simulink model "power_wind"  (R2014b)
settings: Solver=ode23tb  StartTime=0.0  StopTime=20  MaxStep=1/60  RelTol=1e-4  AbsTol=1e-3
InitFcn:
  | xInitial = init_power_wind_ig;
undefined symbols (not defined in the file): D1, D11, Delta
libraries: powerlib_meascontrol x45, powerlib x29, DRlib x3, factslib x1
(part 3 of 4)

== system power_wind/Wind Farm/Wind Turbine Protections/Protection System3/AC Voltage Protection/Voltage Measurement/magnitude1 ==
  In1 : Inport
  Complex to Real-Imag : ComplexToRealImag
  Fourier1 : Subsystem  mask(Fourier analyser){f1=Freq, n=0}
      mask prompts: f1 "Fundamental frequency f1 (Hz):"; n "Harmonic n (0=DC; 1=fundamental; 2=2nd harm;  ...) :"
      mask help: The Fourier block performs a Fourier analysis of the input signal over a running window of one cycle of the fundamental frequency. First and second outputs return respectively the magnitude and phase (degrees) of the harmonic component specified.
      mask init:
      | k=2-(n==0);
      mask Help: helpview(psbhelp)
  Fourier2 : Subsystem  mask(Fourier analyser){f1=Freq, n=0}
      mask prompts: f1 "Fundamental frequency f1 (Hz):"; n "Harmonic n (0=DC; 1=fundamental; 2=2nd harm;  ...) :"
      mask help: The Fourier block performs a Fourier analysis of the input signal over a running window of one cycle of the fundamental frequency. First and second outputs return respectively the magnitude and phase (degrees) of the harmonic component specified.
      mask init:
      | k=2-(n==0);
      mask Help: helpview(psbhelp)
  Math Function : Math  Operator=hypot  SaturateOnIntegerOverflow=on
  Terminator : Terminator
  Terminator1 : Terminator
  Out1 : Outport
  wires:
  Complex to Real-Imag/1 -> Fourier1/1(signal)
  Complex to Real-Imag/2 -> Fourier2/1(signal)
  Fourier1/2(angle) -> Terminator/1
  Fourier2/2(angle) -> Terminator1/1
  Fourier1/1(magnitude) -> Math Function/1
  Fourier2/1(magnitude) -> Math Function/2
  Math Function/1 -> Out1/1
  In1/1 -> Complex to Real-Imag/1

== system power_wind/Wind Farm/Wind Turbine Protections/Protection System3/AC Voltage Protection/Voltage Measurement/magnitude2 ==
  In1 : Inport
  Complex to Real-Imag : ComplexToRealImag
  Fourier1 : Subsystem  mask(Fourier analyser){f1=Freq, n=0}
      mask prompts: f1 "Fundamental frequency f1 (Hz):"; n "Harmonic n (0=DC; 1=fundamental; 2=2nd harm;  ...) :"
      mask help: The Fourier block performs a Fourier analysis of the input signal over a running window of one cycle of the fundamental frequency. First and second outputs return respectively the magnitude and phase (degrees) of the harmonic component specified.
      mask init:
      | k=2-(n==0);
      mask Help: helpview(psbhelp)
  Fourier2 : Subsystem  mask(Fourier analyser){f1=Freq, n=0}
      mask prompts: f1 "Fundamental frequency f1 (Hz):"; n "Harmonic n (0=DC; 1=fundamental; 2=2nd harm;  ...) :"
      mask help: The Fourier block performs a Fourier analysis of the input signal over a running window of one cycle of the fundamental frequency. First and second outputs return respectively the magnitude and phase (degrees) of the harmonic component specified.
      mask init:
      | k=2-(n==0);
      mask Help: helpview(psbhelp)
  Math Function : Math  Operator=hypot  SaturateOnIntegerOverflow=on
  Terminator : Terminator
  Terminator1 : Terminator
  Out1 : Outport
  wires:
  In1/1 -> Complex to Real-Imag/1
  Math Function/1 -> Out1/1
  Fourier2/1(magnitude) -> Math Function/2
  Fourier1/1(magnitude) -> Math Function/1
  Fourier2/2(angle) -> Terminator1/1
  Fourier1/2(angle) -> Terminator/1
  Complex to Real-Imag/2 -> Fourier2/1(signal)
  Complex to Real-Imag/1 -> Fourier1/1(signal)

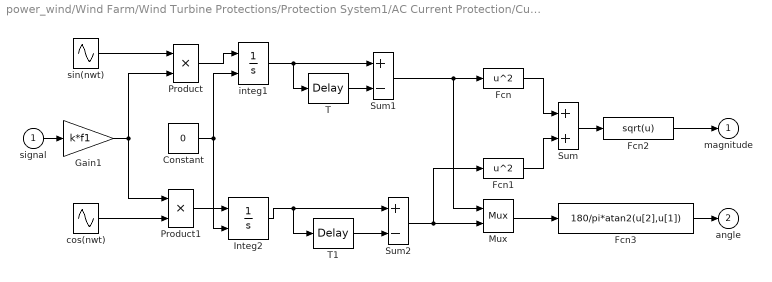
== system power_wind/Wind Farm/Wind Turbine Protections/Protection System1/AC Current Protection/Current Measurement/magnitude/Fourier1 ==
  signal : Inport
  Constant : Constant  Value=0
  Fcn : Fcn  Expr=u^2
  Fcn1 : Fcn  Expr=u^2
  Fcn2 : Fcn  Expr=sqrt(u)
  Fcn3 : Fcn  Expr=180/pi*atan2(u[2],u[1])
  Gain1 : Gain  Gain=k*f1  SaturateOnIntegerOverflow=on  OutDataTypeStr=Inherit: Same as input  ParamDataTypeStr=Inherit: Same as input
  Integ2 : Integrator  InitialConditionSource=external
  Mux : Mux  Inputs=2
  Product : Product  SaturateOnIntegerOverflow=on  InputSameDT=on  OutDataTypeStr=Inherit: Same as first input
  Product1 : Product  SaturateOnIntegerOverflow=on  InputSameDT=on  OutDataTypeStr=Inherit: Same as first input
  Sum : Sum  SaturateOnIntegerOverflow=on  InputSameDT=on  OutDataTypeStr=Inherit: Same as first input
  Sum1 : Sum  Inputs=+-  SaturateOnIntegerOverflow=on  InputSameDT=on  OutDataTypeStr=Inherit: Same as first input
  Sum2 : Sum  Inputs=+-  SaturateOnIntegerOverflow=on  InputSameDT=on  OutDataTypeStr=Inherit: Same as first input
  T : TransportDelay  DelayTime=1/f1  BufferSize=2048
  T1 : TransportDelay  DelayTime=1/f1  BufferSize=2048
  cos(nwt) : Sin  Frequency=2*pi*n*f1  Phase=pi/2  SampleTime=0
  integ1 : Integrator  InitialConditionSource=external
  sin(nwt) : Sin  Frequency=2*pi*n*f1  SampleTime=0
  magnitude : Outport  InitialOutput=0
  angle : Outport  Port=2  InitialOutput=0
  wires:
  Constant/1 -> integ1/2, Integ2/2
  Sum/1 -> Fcn2/1
  Fcn/1 -> Sum/1
  Fcn1/1 -> Sum/2
  Mux/1 -> Fcn3/1
  Fcn3/1 -> angle/1
  sin(nwt)/1 -> Product/1
  cos(nwt)/1 -> Product1/2
  Product/1 -> integ1/1
  Product1/1 -> Integ2/1
  T/1 -> Sum1/2
  T1/1 -> Sum2/2
  integ1/1 -> Sum1/1, T/1
  Integ2/1 -> T1/1, Sum2/1
  Sum2/1 -> Fcn1/1, Mux/2
  Sum1/1 -> Fcn/1, Mux/1
  signal/1 -> Gain1/1
  Gain1/1 -> Product/2, Product1/1
  Fcn2/1 -> magnitude/1

== system power_wind/Wind Farm/Wind Turbine Protections/Protection System1/AC Current Protection/Current Measurement/magnitude/Fourier2 ==
  signal : Inport
  Constant : Constant  Value=0
  Fcn : Fcn  Expr=u^2
  Fcn1 : Fcn  Expr=u^2
  Fcn2 : Fcn  Expr=sqrt(u)
  Fcn3 : Fcn  Expr=180/pi*atan2(u[2],u[1])
  Gain1 : Gain  Gain=k*f1  SaturateOnIntegerOverflow=on  OutDataTypeStr=Inherit: Same as input  ParamDataTypeStr=Inherit: Same as input
  Integ2 : Integrator  InitialConditionSource=external
  Mux : Mux  Inputs=2
  Product : Product  SaturateOnIntegerOverflow=on  InputSameDT=on  OutDataTypeStr=Inherit: Same as first input
  Product1 : Product  SaturateOnIntegerOverflow=on  InputSameDT=on  OutDataTypeStr=Inherit: Same as first input
  Sum : Sum  SaturateOnIntegerOverflow=on  InputSameDT=on  OutDataTypeStr=Inherit: Same as first input
  Sum1 : Sum  Inputs=+-  SaturateOnIntegerOverflow=on  InputSameDT=on  OutDataTypeStr=Inherit: Same as first input
  Sum2 : Sum  Inputs=+-  SaturateOnIntegerOverflow=on  InputSameDT=on  OutDataTypeStr=Inherit: Same as first input
  T : TransportDelay  DelayTime=1/f1  BufferSize=2048
  T1 : TransportDelay  DelayTime=1/f1  BufferSize=2048
  cos(nwt) : Sin  Frequency=2*pi*n*f1  Phase=pi/2  SampleTime=0
  integ1 : Integrator  InitialConditionSource=external
  sin(nwt) : Sin  Frequency=2*pi*n*f1  SampleTime=0
  magnitude : Outport  InitialOutput=0
  angle : Outport  Port=2  InitialOutput=0
  wires:
  Fcn2/1 -> magnitude/1
  Gain1/1 -> Product1/1, Product/2
  signal/1 -> Gain1/1
  Sum1/1 -> Mux/1, Fcn/1
  Sum2/1 -> Mux/2, Fcn1/1
  Integ2/1 -> Sum2/1, T1/1
  integ1/1 -> T/1, Sum1/1
  T1/1 -> Sum2/2
  T/1 -> Sum1/2
  Product1/1 -> Integ2/1
  Product/1 -> integ1/1
  cos(nwt)/1 -> Product1/2
  sin(nwt)/1 -> Product/1
  Fcn3/1 -> angle/1
  Mux/1 -> Fcn3/1
  Fcn1/1 -> Sum/2
  Fcn/1 -> Sum/1
  Sum/1 -> Fcn2/1
  Constant/1 -> Integ2/2, integ1/2

== system power_wind/Wind Farm/Wind Turbine Protections/Protection System1/AC Current Protection/Current Measurement/magnitude1/Fourier1 ==
  signal : Inport
  Constant : Constant  Value=0
  Fcn : Fcn  Expr=u^2
  Fcn1 : Fcn  Expr=u^2
  Fcn2 : Fcn  Expr=sqrt(u)
  Fcn3 : Fcn  Expr=180/pi*atan2(u[2],u[1])
  Gain1 : Gain  Gain=k*f1  SaturateOnIntegerOverflow=on  OutDataTypeStr=Inherit: Same as input  ParamDataTypeStr=Inherit: Same as input
  Integ2 : Integrator  InitialConditionSource=external
  Mux : Mux  Inputs=2
  Product : Product  SaturateOnIntegerOverflow=on  InputSameDT=on  OutDataTypeStr=Inherit: Same as first input
  Product1 : Product  SaturateOnIntegerOverflow=on  InputSameDT=on  OutDataTypeStr=Inherit: Same as first input
  Sum : Sum  SaturateOnIntegerOverflow=on  InputSameDT=on  OutDataTypeStr=Inherit: Same as first input
  Sum1 : Sum  Inputs=+-  SaturateOnIntegerOverflow=on  InputSameDT=on  OutDataTypeStr=Inherit: Same as first input
  Sum2 : Sum  Inputs=+-  SaturateOnIntegerOverflow=on  InputSameDT=on  OutDataTypeStr=Inherit: Same as first input
  T : TransportDelay  DelayTime=1/f1  BufferSize=2048
  T1 : TransportDelay  DelayTime=1/f1  BufferSize=2048
  cos(nwt) : Sin  Frequency=2*pi*n*f1  Phase=pi/2  SampleTime=0
  integ1 : Integrator  InitialConditionSource=external
  sin(nwt) : Sin  Frequency=2*pi*n*f1  SampleTime=0
  magnitude : Outport  InitialOutput=0
  angle : Outport  Port=2  InitialOutput=0
  wires:
  Fcn2/1 -> magnitude/1
  Gain1/1 -> Product1/1, Product/2
  signal/1 -> Gain1/1
  Sum1/1 -> Mux/1, Fcn/1
  Sum2/1 -> Mux/2, Fcn1/1
  Integ2/1 -> Sum2/1, T1/1
  integ1/1 -> T/1, Sum1/1
  T1/1 -> Sum2/2
  T/1 -> Sum1/2
  Product1/1 -> Integ2/1
  Product/1 -> integ1/1
  cos(nwt)/1 -> Product1/2
  sin(nwt)/1 -> Product/1
  Fcn3/1 -> angle/1
  Mux/1 -> Fcn3/1
  Fcn1/1 -> Sum/2
  Fcn/1 -> Sum/1
  Sum/1 -> Fcn2/1
  Constant/1 -> Integ2/2, integ1/2

== system power_wind/Wind Farm/Wind Turbine Protections/Protection System1/AC Current Protection/Current Measurement/magnitude1/Fourier2 ==
  signal : Inport
  Constant : Constant  Value=0
  Fcn : Fcn  Expr=u^2
  Fcn1 : Fcn  Expr=u^2
  Fcn2 : Fcn  Expr=sqrt(u)
  Fcn3 : Fcn  Expr=180/pi*atan2(u[2],u[1])
  Gain1 : Gain  Gain=k*f1  SaturateOnIntegerOverflow=on  OutDataTypeStr=Inherit: Same as input  ParamDataTypeStr=Inherit: Same as input
  Integ2 : Integrator  InitialConditionSource=external
  Mux : Mux  Inputs=2
  Product : Product  SaturateOnIntegerOverflow=on  InputSameDT=on  OutDataTypeStr=Inherit: Same as first input
  Product1 : Product  SaturateOnIntegerOverflow=on  InputSameDT=on  OutDataTypeStr=Inherit: Same as first input
  Sum : Sum  SaturateOnIntegerOverflow=on  InputSameDT=on  OutDataTypeStr=Inherit: Same as first input
  Sum1 : Sum  Inputs=+-  SaturateOnIntegerOverflow=on  InputSameDT=on  OutDataTypeStr=Inherit: Same as first input
  Sum2 : Sum  Inputs=+-  SaturateOnIntegerOverflow=on  InputSameDT=on  OutDataTypeStr=Inherit: Same as first input
  T : TransportDelay  DelayTime=1/f1  BufferSize=2048
  T1 : TransportDelay  DelayTime=1/f1  BufferSize=2048
  cos(nwt) : Sin  Frequency=2*pi*n*f1  Phase=pi/2  SampleTime=0
  integ1 : Integrator  InitialConditionSource=external
  sin(nwt) : Sin  Frequency=2*pi*n*f1  SampleTime=0
  magnitude : Outport  InitialOutput=0
  angle : Outport  Port=2  InitialOutput=0
  wires:
  Constant/1 -> integ1/2, Integ2/2
  Sum/1 -> Fcn2/1
  Fcn/1 -> Sum/1
  Fcn1/1 -> Sum/2
  Mux/1 -> Fcn3/1
  Fcn3/1 -> angle/1
  sin(nwt)/1 -> Product/1
  cos(nwt)/1 -> Product1/2
  Product/1 -> integ1/1
  Product1/1 -> Integ2/1
  T/1 -> Sum1/2
  T1/1 -> Sum2/2
  integ1/1 -> Sum1/1, T/1
  Integ2/1 -> T1/1, Sum2/1
  Sum2/1 -> Fcn1/1, Mux/2
  Sum1/1 -> Fcn/1, Mux/1
  signal/1 -> Gain1/1
  Gain1/1 -> Product/2, Product1/1
  Fcn2/1 -> magnitude/1

== system power_wind/Wind Farm/Wind Turbine Protections/Protection System1/AC Voltage Protection/Voltage Measurement/magnitude/Fourier1 ==
  signal : Inport
  Constant : Constant  Value=0
  Fcn : Fcn  Expr=u^2
  Fcn1 : Fcn  Expr=u^2
  Fcn2 : Fcn  Expr=sqrt(u)
  Fcn3 : Fcn  Expr=180/pi*atan2(u[2],u[1])
  Gain1 : Gain  Gain=k*f1  SaturateOnIntegerOverflow=on  OutDataTypeStr=Inherit: Same as input  ParamDataTypeStr=Inherit: Same as input
  Integ2 : Integrator  InitialConditionSource=external
  Mux : Mux  Inputs=2
  Product : Product  SaturateOnIntegerOverflow=on  InputSameDT=on  OutDataTypeStr=Inherit: Same as first input
  Product1 : Product  SaturateOnIntegerOverflow=on  InputSameDT=on  OutDataTypeStr=Inherit: Same as first input
  Sum : Sum  SaturateOnIntegerOverflow=on  InputSameDT=on  OutDataTypeStr=Inherit: Same as first input
  Sum1 : Sum  Inputs=+-  SaturateOnIntegerOverflow=on  InputSameDT=on  OutDataTypeStr=Inherit: Same as first input
  Sum2 : Sum  Inputs=+-  SaturateOnIntegerOverflow=on  InputSameDT=on  OutDataTypeStr=Inherit: Same as first input
  T : TransportDelay  DelayTime=1/f1  BufferSize=2048
  T1 : TransportDelay  DelayTime=1/f1  BufferSize=2048
  cos(nwt) : Sin  Frequency=2*pi*n*f1  Phase=pi/2  SampleTime=0
  integ1 : Integrator  InitialConditionSource=external
  sin(nwt) : Sin  Frequency=2*pi*n*f1  SampleTime=0
  magnitude : Outport  InitialOutput=0
  angle : Outport  Port=2  InitialOutput=0
  wires:
  Constant/1 -> integ1/2, Integ2/2
  Sum/1 -> Fcn2/1
  Fcn/1 -> Sum/1
  Fcn1/1 -> Sum/2
  Mux/1 -> Fcn3/1
  Fcn3/1 -> angle/1
  sin(nwt)/1 -> Product/1
  cos(nwt)/1 -> Product1/2
  Product/1 -> integ1/1
  Product1/1 -> Integ2/1
  T/1 -> Sum1/2
  T1/1 -> Sum2/2
  integ1/1 -> Sum1/1, T/1
  Integ2/1 -> T1/1, Sum2/1
  Sum2/1 -> Fcn1/1, Mux/2
  Sum1/1 -> Fcn/1, Mux/1
  signal/1 -> Gain1/1
  Gain1/1 -> Product/2, Product1/1
  Fcn2/1 -> magnitude/1

== system power_wind/Wind Farm/Wind Turbine Protections/Protection System1/AC Voltage Protection/Voltage Measurement/magnitude/Fourier2 ==
  signal : Inport
  Constant : Constant  Value=0
  Fcn : Fcn  Expr=u^2
  Fcn1 : Fcn  Expr=u^2
  Fcn2 : Fcn  Expr=sqrt(u)
  Fcn3 : Fcn  Expr=180/pi*atan2(u[2],u[1])
  Gain1 : Gain  Gain=k*f1  SaturateOnIntegerOverflow=on  OutDataTypeStr=Inherit: Same as input  ParamDataTypeStr=Inherit: Same as input
  Integ2 : Integrator  InitialConditionSource=external
  Mux : Mux  Inputs=2
  Product : Product  SaturateOnIntegerOverflow=on  InputSameDT=on  OutDataTypeStr=Inherit: Same as first input
  Product1 : Product  SaturateOnIntegerOverflow=on  InputSameDT=on  OutDataTypeStr=Inherit: Same as first input
  Sum : Sum  SaturateOnIntegerOverflow=on  InputSameDT=on  OutDataTypeStr=Inherit: Same as first input
  Sum1 : Sum  Inputs=+-  SaturateOnIntegerOverflow=on  InputSameDT=on  OutDataTypeStr=Inherit: Same as first input
  Sum2 : Sum  Inputs=+-  SaturateOnIntegerOverflow=on  InputSameDT=on  OutDataTypeStr=Inherit: Same as first input
  T : TransportDelay  DelayTime=1/f1  BufferSize=2048
  T1 : TransportDelay  DelayTime=1/f1  BufferSize=2048
  cos(nwt) : Sin  Frequency=2*pi*n*f1  Phase=pi/2  SampleTime=0
  integ1 : Integrator  InitialConditionSource=external
  sin(nwt) : Sin  Frequency=2*pi*n*f1  SampleTime=0
  magnitude : Outport  InitialOutput=0
  angle : Outport  Port=2  InitialOutput=0
  wires:
  Fcn2/1 -> magnitude/1
  Gain1/1 -> Product1/1, Product/2
  signal/1 -> Gain1/1
  Sum1/1 -> Mux/1, Fcn/1
  Sum2/1 -> Mux/2, Fcn1/1
  Integ2/1 -> Sum2/1, T1/1
  integ1/1 -> T/1, Sum1/1
  T1/1 -> Sum2/2
  T/1 -> Sum1/2
  Product1/1 -> Integ2/1
  Product/1 -> integ1/1
  cos(nwt)/1 -> Product1/2
  sin(nwt)/1 -> Product/1
  Fcn3/1 -> angle/1
  Mux/1 -> Fcn3/1
  Fcn1/1 -> Sum/2
  Fcn/1 -> Sum/1
  Sum/1 -> Fcn2/1
  Constant/1 -> Integ2/2, integ1/2

== system power_wind/Wind Farm/Wind Turbine Protections/Protection System1/AC Voltage Protection/Voltage Measurement/magnitude1/Fourier1 ==
  signal : Inport
  Constant : Constant  Value=0
  Fcn : Fcn  Expr=u^2
  Fcn1 : Fcn  Expr=u^2
  Fcn2 : Fcn  Expr=sqrt(u)
  Fcn3 : Fcn  Expr=180/pi*atan2(u[2],u[1])
  Gain1 : Gain  Gain=k*f1  SaturateOnIntegerOverflow=on  OutDataTypeStr=Inherit: Same as input  ParamDataTypeStr=Inherit: Same as input
  Integ2 : Integrator  InitialConditionSource=external
  Mux : Mux  Inputs=2
  Product : Product  SaturateOnIntegerOverflow=on  InputSameDT=on  OutDataTypeStr=Inherit: Same as first input
  Product1 : Product  SaturateOnIntegerOverflow=on  InputSameDT=on  OutDataTypeStr=Inherit: Same as first input
  Sum : Sum  SaturateOnIntegerOverflow=on  InputSameDT=on  OutDataTypeStr=Inherit: Same as first input
  Sum1 : Sum  Inputs=+-  SaturateOnIntegerOverflow=on  InputSameDT=on  OutDataTypeStr=Inherit: Same as first input
  Sum2 : Sum  Inputs=+-  SaturateOnIntegerOverflow=on  InputSameDT=on  OutDataTypeStr=Inherit: Same as first input
  T : TransportDelay  DelayTime=1/f1  BufferSize=2048
  T1 : TransportDelay  DelayTime=1/f1  BufferSize=2048
  cos(nwt) : Sin  Frequency=2*pi*n*f1  Phase=pi/2  SampleTime=0
  integ1 : Integrator  InitialConditionSource=external
  sin(nwt) : Sin  Frequency=2*pi*n*f1  SampleTime=0
  magnitude : Outport  InitialOutput=0
  angle : Outport  Port=2  InitialOutput=0
  wires:
  Fcn2/1 -> magnitude/1
  Gain1/1 -> Product1/1, Product/2
  signal/1 -> Gain1/1
  Sum1/1 -> Mux/1, Fcn/1
  Sum2/1 -> Mux/2, Fcn1/1
  Integ2/1 -> Sum2/1, T1/1
  integ1/1 -> T/1, Sum1/1
  T1/1 -> Sum2/2
  T/1 -> Sum1/2
  Product1/1 -> Integ2/1
  Product/1 -> integ1/1
  cos(nwt)/1 -> Product1/2
  sin(nwt)/1 -> Product/1
  Fcn3/1 -> angle/1
  Mux/1 -> Fcn3/1
  Fcn1/1 -> Sum/2
  Fcn/1 -> Sum/1
  Sum/1 -> Fcn2/1
  Constant/1 -> Integ2/2, integ1/2

== system power_wind/Wind Farm/Wind Turbine Protections/Protection System1/AC Voltage Protection/Voltage Measurement/magnitude1/Fourier2 ==
  signal : Inport
  Constant : Constant  Value=0
  Fcn : Fcn  Expr=u^2
  Fcn1 : Fcn  Expr=u^2
  Fcn2 : Fcn  Expr=sqrt(u)
  Fcn3 : Fcn  Expr=180/pi*atan2(u[2],u[1])
  Gain1 : Gain  Gain=k*f1  SaturateOnIntegerOverflow=on  OutDataTypeStr=Inherit: Same as input  ParamDataTypeStr=Inherit: Same as input
  Integ2 : Integrator  InitialConditionSource=external
  Mux : Mux  Inputs=2
  Product : Product  SaturateOnIntegerOverflow=on  InputSameDT=on  OutDataTypeStr=Inherit: Same as first input
  Product1 : Product  SaturateOnIntegerOverflow=on  InputSameDT=on  OutDataTypeStr=Inherit: Same as first input
  Sum : Sum  SaturateOnIntegerOverflow=on  InputSameDT=on  OutDataTypeStr=Inherit: Same as first input
  Sum1 : Sum  Inputs=+-  SaturateOnIntegerOverflow=on  InputSameDT=on  OutDataTypeStr=Inherit: Same as first input
  Sum2 : Sum  Inputs=+-  SaturateOnIntegerOverflow=on  InputSameDT=on  OutDataTypeStr=Inherit: Same as first input
  T : TransportDelay  DelayTime=1/f1  BufferSize=2048
  T1 : TransportDelay  DelayTime=1/f1  BufferSize=2048
  cos(nwt) : Sin  Frequency=2*pi*n*f1  Phase=pi/2  SampleTime=0
  integ1 : Integrator  InitialConditionSource=external
  sin(nwt) : Sin  Frequency=2*pi*n*f1  SampleTime=0
  magnitude : Outport  InitialOutput=0
  angle : Outport  Port=2  InitialOutput=0
  wires:
  Constant/1 -> integ1/2, Integ2/2
  Sum/1 -> Fcn2/1
  Fcn/1 -> Sum/1
  Fcn1/1 -> Sum/2
  Mux/1 -> Fcn3/1
  Fcn3/1 -> angle/1
  sin(nwt)/1 -> Product/1
  cos(nwt)/1 -> Product1/2
  Product/1 -> integ1/1
  Product1/1 -> Integ2/1
  T/1 -> Sum1/2
  T1/1 -> Sum2/2
  integ1/1 -> Sum1/1, T/1
  Integ2/1 -> T1/1, Sum2/1
  Sum2/1 -> Fcn1/1, Mux/2
  Sum1/1 -> Fcn/1, Mux/1
  signal/1 -> Gain1/1
  Gain1/1 -> Product/2, Product1/1
  Fcn2/1 -> magnitude/1

== system power_wind/Wind Farm/Wind Turbine Protections/Protection System1/AC Voltage Protection/Voltage Measurement/magnitude2/Fourier1 ==
  signal : Inport
  Constant : Constant  Value=0
  Fcn : Fcn  Expr=u^2
  Fcn1 : Fcn  Expr=u^2
  Fcn2 : Fcn  Expr=sqrt(u)
  Fcn3 : Fcn  Expr=180/pi*atan2(u[2],u[1])
  Gain1 : Gain  Gain=k*f1  SaturateOnIntegerOverflow=on  OutDataTypeStr=Inherit: Same as input  ParamDataTypeStr=Inherit: Same as input
  Integ2 : Integrator  InitialConditionSource=external
  Mux : Mux  Inputs=2
  Product : Product  SaturateOnIntegerOverflow=on  InputSameDT=on  OutDataTypeStr=Inherit: Same as first input
  Product1 : Product  SaturateOnIntegerOverflow=on  InputSameDT=on  OutDataTypeStr=Inherit: Same as first input
  Sum : Sum  SaturateOnIntegerOverflow=on  InputSameDT=on  OutDataTypeStr=Inherit: Same as first input
  Sum1 : Sum  Inputs=+-  SaturateOnIntegerOverflow=on  InputSameDT=on  OutDataTypeStr=Inherit: Same as first input
  Sum2 : Sum  Inputs=+-  SaturateOnIntegerOverflow=on  InputSameDT=on  OutDataTypeStr=Inherit: Same as first input
  T : TransportDelay  DelayTime=1/f1  BufferSize=2048
  T1 : TransportDelay  DelayTime=1/f1  BufferSize=2048
  cos(nwt) : Sin  Frequency=2*pi*n*f1  Phase=pi/2  SampleTime=0
  integ1 : Integrator  InitialConditionSource=external
  sin(nwt) : Sin  Frequency=2*pi*n*f1  SampleTime=0
  magnitude : Outport  InitialOutput=0
  angle : Outport  Port=2  InitialOutput=0
  wires:
  Constant/1 -> integ1/2, Integ2/2
  Sum/1 -> Fcn2/1
  Fcn/1 -> Sum/1
  Fcn1/1 -> Sum/2
  Mux/1 -> Fcn3/1
  Fcn3/1 -> angle/1
  sin(nwt)/1 -> Product/1
  cos(nwt)/1 -> Product1/2
  Product/1 -> integ1/1
  Product1/1 -> Integ2/1
  T/1 -> Sum1/2
  T1/1 -> Sum2/2
  integ1/1 -> Sum1/1, T/1
  Integ2/1 -> T1/1, Sum2/1
  Sum2/1 -> Fcn1/1, Mux/2
  Sum1/1 -> Fcn/1, Mux/1
  signal/1 -> Gain1/1
  Gain1/1 -> Product/2, Product1/1
  Fcn2/1 -> magnitude/1

== system power_wind/Wind Farm/Wind Turbine Protections/Protection System1/AC Voltage Protection/Voltage Measurement/magnitude2/Fourier2 ==
  signal : Inport
  Constant : Constant  Value=0
  Fcn : Fcn  Expr=u^2
  Fcn1 : Fcn  Expr=u^2
  Fcn2 : Fcn  Expr=sqrt(u)
  Fcn3 : Fcn  Expr=180/pi*atan2(u[2],u[1])
  Gain1 : Gain  Gain=k*f1  SaturateOnIntegerOverflow=on  OutDataTypeStr=Inherit: Same as input  ParamDataTypeStr=Inherit: Same as input
  Integ2 : Integrator  InitialConditionSource=external
  Mux : Mux  Inputs=2
  Product : Product  SaturateOnIntegerOverflow=on  InputSameDT=on  OutDataTypeStr=Inherit: Same as first input
  Product1 : Product  SaturateOnIntegerOverflow=on  InputSameDT=on  OutDataTypeStr=Inherit: Same as first input
  Sum : Sum  SaturateOnIntegerOverflow=on  InputSameDT=on  OutDataTypeStr=Inherit: Same as first input
  Sum1 : Sum  Inputs=+-  SaturateOnIntegerOverflow=on  InputSameDT=on  OutDataTypeStr=Inherit: Same as first input
  Sum2 : Sum  Inputs=+-  SaturateOnIntegerOverflow=on  InputSameDT=on  OutDataTypeStr=Inherit: Same as first input
  T : TransportDelay  DelayTime=1/f1  BufferSize=2048
  T1 : TransportDelay  DelayTime=1/f1  BufferSize=2048
  cos(nwt) : Sin  Frequency=2*pi*n*f1  Phase=pi/2  SampleTime=0
  integ1 : Integrator  InitialConditionSource=external
  sin(nwt) : Sin  Frequency=2*pi*n*f1  SampleTime=0
  magnitude : Outport  InitialOutput=0
  angle : Outport  Port=2  InitialOutput=0
  wires:
  Fcn2/1 -> magnitude/1
  Gain1/1 -> Product1/1, Product/2
  signal/1 -> Gain1/1
  Sum1/1 -> Mux/1, Fcn/1
  Sum2/1 -> Mux/2, Fcn1/1
  Integ2/1 -> Sum2/1, T1/1
  integ1/1 -> T/1, Sum1/1
  T1/1 -> Sum2/2
  T/1 -> Sum1/2
  Product1/1 -> Integ2/1
  Product/1 -> integ1/1
  cos(nwt)/1 -> Product1/2
  sin(nwt)/1 -> Product/1
  Fcn3/1 -> angle/1
  Mux/1 -> Fcn3/1
  Fcn1/1 -> Sum/2
  Fcn/1 -> Sum/1
  Sum/1 -> Fcn2/1
  Constant/1 -> Integ2/2, integ1/2

== system power_wind/Wind Farm/Wind Turbine Protections/Protection System2/AC Current Protection/Current Measurement/magnitude/Fourier1 ==
  signal : Inport
  Constant : Constant  Value=0
  Fcn : Fcn  Expr=u^2
  Fcn1 : Fcn  Expr=u^2
  Fcn2 : Fcn  Expr=sqrt(u)
  Fcn3 : Fcn  Expr=180/pi*atan2(u[2],u[1])
  Gain1 : Gain  Gain=k*f1  SaturateOnIntegerOverflow=on  OutDataTypeStr=Inherit: Same as input  ParamDataTypeStr=Inherit: Same as input
  Integ2 : Integrator  InitialConditionSource=external
  Mux : Mux  Inputs=2
  Product : Product  SaturateOnIntegerOverflow=on  InputSameDT=on  OutDataTypeStr=Inherit: Same as first input
  Product1 : Product  SaturateOnIntegerOverflow=on  InputSameDT=on  OutDataTypeStr=Inherit: Same as first input
  Sum : Sum  SaturateOnIntegerOverflow=on  InputSameDT=on  OutDataTypeStr=Inherit: Same as first input
  Sum1 : Sum  Inputs=+-  SaturateOnIntegerOverflow=on  InputSameDT=on  OutDataTypeStr=Inherit: Same as first input
  Sum2 : Sum  Inputs=+-  SaturateOnIntegerOverflow=on  InputSameDT=on  OutDataTypeStr=Inherit: Same as first input
  T : TransportDelay  DelayTime=1/f1  BufferSize=2048
  T1 : TransportDelay  DelayTime=1/f1  BufferSize=2048
  cos(nwt) : Sin  Frequency=2*pi*n*f1  Phase=pi/2  SampleTime=0
  integ1 : Integrator  InitialConditionSource=external
  sin(nwt) : Sin  Frequency=2*pi*n*f1  SampleTime=0
  magnitude : Outport  InitialOutput=0
  angle : Outport  Port=2  InitialOutput=0
  wires:
  Fcn2/1 -> magnitude/1
  Gain1/1 -> Product1/1, Product/2
  signal/1 -> Gain1/1
  Sum1/1 -> Mux/1, Fcn/1
  Sum2/1 -> Mux/2, Fcn1/1
  Integ2/1 -> Sum2/1, T1/1
  integ1/1 -> T/1, Sum1/1
  T1/1 -> Sum2/2
  T/1 -> Sum1/2
  Product1/1 -> Integ2/1
  Product/1 -> integ1/1
  cos(nwt)/1 -> Product1/2
  sin(nwt)/1 -> Product/1
  Fcn3/1 -> angle/1
  Mux/1 -> Fcn3/1
  Fcn1/1 -> Sum/2
  Fcn/1 -> Sum/1
  Sum/1 -> Fcn2/1
  Constant/1 -> Integ2/2, integ1/2

== system power_wind/Wind Farm/Wind Turbine Protections/Protection System2/AC Current Protection/Current Measurement/magnitude/Fourier2 ==
  signal : Inport
  Constant : Constant  Value=0
  Fcn : Fcn  Expr=u^2
  Fcn1 : Fcn  Expr=u^2
  Fcn2 : Fcn  Expr=sqrt(u)
  Fcn3 : Fcn  Expr=180/pi*atan2(u[2],u[1])
  Gain1 : Gain  Gain=k*f1  SaturateOnIntegerOverflow=on  OutDataTypeStr=Inherit: Same as input  ParamDataTypeStr=Inherit: Same as input
  Integ2 : Integrator  InitialConditionSource=external
  Mux : Mux  Inputs=2
  Product : Product  SaturateOnIntegerOverflow=on  InputSameDT=on  OutDataTypeStr=Inherit: Same as first input
  Product1 : Product  SaturateOnIntegerOverflow=on  InputSameDT=on  OutDataTypeStr=Inherit: Same as first input
  Sum : Sum  SaturateOnIntegerOverflow=on  InputSameDT=on  OutDataTypeStr=Inherit: Same as first input
  Sum1 : Sum  Inputs=+-  SaturateOnIntegerOverflow=on  InputSameDT=on  OutDataTypeStr=Inherit: Same as first input
  Sum2 : Sum  Inputs=+-  SaturateOnIntegerOverflow=on  InputSameDT=on  OutDataTypeStr=Inherit: Same as first input
  T : TransportDelay  DelayTime=1/f1  BufferSize=2048
  T1 : TransportDelay  DelayTime=1/f1  BufferSize=2048
  cos(nwt) : Sin  Frequency=2*pi*n*f1  Phase=pi/2  SampleTime=0
  integ1 : Integrator  InitialConditionSource=external
  sin(nwt) : Sin  Frequency=2*pi*n*f1  SampleTime=0
  magnitude : Outport  InitialOutput=0
  angle : Outport  Port=2  InitialOutput=0
  wires:
  Constant/1 -> integ1/2, Integ2/2
  Sum/1 -> Fcn2/1
  Fcn/1 -> Sum/1
  Fcn1/1 -> Sum/2
  Mux/1 -> Fcn3/1
  Fcn3/1 -> angle/1
  sin(nwt)/1 -> Product/1
  cos(nwt)/1 -> Product1/2
  Product/1 -> integ1/1
  Product1/1 -> Integ2/1
  T/1 -> Sum1/2
  T1/1 -> Sum2/2
  integ1/1 -> Sum1/1, T/1
  Integ2/1 -> T1/1, Sum2/1
  Sum2/1 -> Fcn1/1, Mux/2
  Sum1/1 -> Fcn/1, Mux/1
  signal/1 -> Gain1/1
  Gain1/1 -> Product/2, Product1/1
  Fcn2/1 -> magnitude/1

== system power_wind/Wind Farm/Wind Turbine Protections/Protection System2/AC Current Protection/Current Measurement/magnitude1/Fourier1 ==
  signal : Inport
  Constant : Constant  Value=0
  Fcn : Fcn  Expr=u^2
  Fcn1 : Fcn  Expr=u^2
  Fcn2 : Fcn  Expr=sqrt(u)
  Fcn3 : Fcn  Expr=180/pi*atan2(u[2],u[1])
  Gain1 : Gain  Gain=k*f1  SaturateOnIntegerOverflow=on  OutDataTypeStr=Inherit: Same as input  ParamDataTypeStr=Inherit: Same as input
  Integ2 : Integrator  InitialConditionSource=external
  Mux : Mux  Inputs=2
  Product : Product  SaturateOnIntegerOverflow=on  InputSameDT=on  OutDataTypeStr=Inherit: Same as first input
  Product1 : Product  SaturateOnIntegerOverflow=on  InputSameDT=on  OutDataTypeStr=Inherit: Same as first input
  Sum : Sum  SaturateOnIntegerOverflow=on  InputSameDT=on  OutDataTypeStr=Inherit: Same as first input
  Sum1 : Sum  Inputs=+-  SaturateOnIntegerOverflow=on  InputSameDT=on  OutDataTypeStr=Inherit: Same as first input
  Sum2 : Sum  Inputs=+-  SaturateOnIntegerOverflow=on  InputSameDT=on  OutDataTypeStr=Inherit: Same as first input
  T : TransportDelay  DelayTime=1/f1  BufferSize=2048
  T1 : TransportDelay  DelayTime=1/f1  BufferSize=2048
  cos(nwt) : Sin  Frequency=2*pi*n*f1  Phase=pi/2  SampleTime=0
  integ1 : Integrator  InitialConditionSource=external
  sin(nwt) : Sin  Frequency=2*pi*n*f1  SampleTime=0
  magnitude : Outport  InitialOutput=0
  angle : Outport  Port=2  InitialOutput=0
  wires:
  Constant/1 -> integ1/2, Integ2/2
  Sum/1 -> Fcn2/1
  Fcn/1 -> Sum/1
  Fcn1/1 -> Sum/2
  Mux/1 -> Fcn3/1
  Fcn3/1 -> angle/1
  sin(nwt)/1 -> Product/1
  cos(nwt)/1 -> Product1/2
  Product/1 -> integ1/1
  Product1/1 -> Integ2/1
  T/1 -> Sum1/2
  T1/1 -> Sum2/2
  integ1/1 -> Sum1/1, T/1
  Integ2/1 -> T1/1, Sum2/1
  Sum2/1 -> Fcn1/1, Mux/2
  Sum1/1 -> Fcn/1, Mux/1
  signal/1 -> Gain1/1
  Gain1/1 -> Product/2, Product1/1
  Fcn2/1 -> magnitude/1

== system power_wind/Wind Farm/Wind Turbine Protections/Protection System2/AC Current Protection/Current Measurement/magnitude1/Fourier2 ==
  signal : Inport
  Constant : Constant  Value=0
  Fcn : Fcn  Expr=u^2
  Fcn1 : Fcn  Expr=u^2
  Fcn2 : Fcn  Expr=sqrt(u)
  Fcn3 : Fcn  Expr=180/pi*atan2(u[2],u[1])
  Gain1 : Gain  Gain=k*f1  SaturateOnIntegerOverflow=on  OutDataTypeStr=Inherit: Same as input  ParamDataTypeStr=Inherit: Same as input
  Integ2 : Integrator  InitialConditionSource=external
  Mux : Mux  Inputs=2
  Product : Product  SaturateOnIntegerOverflow=on  InputSameDT=on  OutDataTypeStr=Inherit: Same as first input
  Product1 : Product  SaturateOnIntegerOverflow=on  InputSameDT=on  OutDataTypeStr=Inherit: Same as first input
  Sum : Sum  SaturateOnIntegerOverflow=on  InputSameDT=on  OutDataTypeStr=Inherit: Same as first input
  Sum1 : Sum  Inputs=+-  SaturateOnIntegerOverflow=on  InputSameDT=on  OutDataTypeStr=Inherit: Same as first input
  Sum2 : Sum  Inputs=+-  SaturateOnIntegerOverflow=on  InputSameDT=on  OutDataTypeStr=Inherit: Same as first input
  T : TransportDelay  DelayTime=1/f1  BufferSize=2048
  T1 : TransportDelay  DelayTime=1/f1  BufferSize=2048
  cos(nwt) : Sin  Frequency=2*pi*n*f1  Phase=pi/2  SampleTime=0
  integ1 : Integrator  InitialConditionSource=external
  sin(nwt) : Sin  Frequency=2*pi*n*f1  SampleTime=0
  magnitude : Outport  InitialOutput=0
  angle : Outport  Port=2  InitialOutput=0
  wires:
  Fcn2/1 -> magnitude/1
  Gain1/1 -> Product1/1, Product/2
  signal/1 -> Gain1/1
  Sum1/1 -> Mux/1, Fcn/1
  Sum2/1 -> Mux/2, Fcn1/1
  Integ2/1 -> Sum2/1, T1/1
  integ1/1 -> T/1, Sum1/1
  T1/1 -> Sum2/2
  T/1 -> Sum1/2
  Product1/1 -> Integ2/1
  Product/1 -> integ1/1
  cos(nwt)/1 -> Product1/2
  sin(nwt)/1 -> Product/1
  Fcn3/1 -> angle/1
  Mux/1 -> Fcn3/1
  Fcn1/1 -> Sum/2
  Fcn/1 -> Sum/1
  Sum/1 -> Fcn2/1
  Constant/1 -> Integ2/2, integ1/2

== system power_wind/Wind Farm/Wind Turbine Protections/Protection System2/AC Voltage Protection/Voltage Measurement/magnitude/Fourier1 ==
  signal : Inport
  Constant : Constant  Value=0
  Fcn : Fcn  Expr=u^2
  Fcn1 : Fcn  Expr=u^2
  Fcn2 : Fcn  Expr=sqrt(u)
  Fcn3 : Fcn  Expr=180/pi*atan2(u[2],u[1])
  Gain1 : Gain  Gain=k*f1  SaturateOnIntegerOverflow=on  OutDataTypeStr=Inherit: Same as input  ParamDataTypeStr=Inherit: Same as input
  Integ2 : Integrator  InitialConditionSource=external
  Mux : Mux  Inputs=2
  Product : Product  SaturateOnIntegerOverflow=on  InputSameDT=on  OutDataTypeStr=Inherit: Same as first input
  Product1 : Product  SaturateOnIntegerOverflow=on  InputSameDT=on  OutDataTypeStr=Inherit: Same as first input
  Sum : Sum  SaturateOnIntegerOverflow=on  InputSameDT=on  OutDataTypeStr=Inherit: Same as first input
  Sum1 : Sum  Inputs=+-  SaturateOnIntegerOverflow=on  InputSameDT=on  OutDataTypeStr=Inherit: Same as first input
  Sum2 : Sum  Inputs=+-  SaturateOnIntegerOverflow=on  InputSameDT=on  OutDataTypeStr=Inherit: Same as first input
  T : TransportDelay  DelayTime=1/f1  BufferSize=2048
  T1 : TransportDelay  DelayTime=1/f1  BufferSize=2048
  cos(nwt) : Sin  Frequency=2*pi*n*f1  Phase=pi/2  SampleTime=0
  integ1 : Integrator  InitialConditionSource=external
  sin(nwt) : Sin  Frequency=2*pi*n*f1  SampleTime=0
  magnitude : Outport  InitialOutput=0
  angle : Outport  Port=2  InitialOutput=0
  wires:
  Fcn2/1 -> magnitude/1
  Gain1/1 -> Product1/1, Product/2
  signal/1 -> Gain1/1
  Sum1/1 -> Mux/1, Fcn/1
  Sum2/1 -> Mux/2, Fcn1/1
  Integ2/1 -> Sum2/1, T1/1
  integ1/1 -> T/1, Sum1/1
  T1/1 -> Sum2/2
  T/1 -> Sum1/2
  Product1/1 -> Integ2/1
  Product/1 -> integ1/1
  cos(nwt)/1 -> Product1/2
  sin(nwt)/1 -> Product/1
  Fcn3/1 -> angle/1
  Mux/1 -> Fcn3/1
  Fcn1/1 -> Sum/2
  Fcn/1 -> Sum/1
  Sum/1 -> Fcn2/1
  Constant/1 -> Integ2/2, integ1/2

== system power_wind/Wind Farm/Wind Turbine Protections/Protection System2/AC Voltage Protection/Voltage Measurement/magnitude/Fourier2 ==
  signal : Inport
  Constant : Constant  Value=0
  Fcn : Fcn  Expr=u^2
  Fcn1 : Fcn  Expr=u^2
  Fcn2 : Fcn  Expr=sqrt(u)
  Fcn3 : Fcn  Expr=180/pi*atan2(u[2],u[1])
  Gain1 : Gain  Gain=k*f1  SaturateOnIntegerOverflow=on  OutDataTypeStr=Inherit: Same as input  ParamDataTypeStr=Inherit: Same as input
  Integ2 : Integrator  InitialConditionSource=external
  Mux : Mux  Inputs=2
  Product : Product  SaturateOnIntegerOverflow=on  InputSameDT=on  OutDataTypeStr=Inherit: Same as first input
  Product1 : Product  SaturateOnIntegerOverflow=on  InputSameDT=on  OutDataTypeStr=Inherit: Same as first input
  Sum : Sum  SaturateOnIntegerOverflow=on  InputSameDT=on  OutDataTypeStr=Inherit: Same as first input
  Sum1 : Sum  Inputs=+-  SaturateOnIntegerOverflow=on  InputSameDT=on  OutDataTypeStr=Inherit: Same as first input
  Sum2 : Sum  Inputs=+-  SaturateOnIntegerOverflow=on  InputSameDT=on  OutDataTypeStr=Inherit: Same as first input
  T : TransportDelay  DelayTime=1/f1  BufferSize=2048
  T1 : TransportDelay  DelayTime=1/f1  BufferSize=2048
  cos(nwt) : Sin  Frequency=2*pi*n*f1  Phase=pi/2  SampleTime=0
  integ1 : Integrator  InitialConditionSource=external
  sin(nwt) : Sin  Frequency=2*pi*n*f1  SampleTime=0
  magnitude : Outport  InitialOutput=0
  angle : Outport  Port=2  InitialOutput=0
  wires:
  Constant/1 -> integ1/2, Integ2/2
  Sum/1 -> Fcn2/1
  Fcn/1 -> Sum/1
  Fcn1/1 -> Sum/2
  Mux/1 -> Fcn3/1
  Fcn3/1 -> angle/1
  sin(nwt)/1 -> Product/1
  cos(nwt)/1 -> Product1/2
  Product/1 -> integ1/1
  Product1/1 -> Integ2/1
  T/1 -> Sum1/2
  T1/1 -> Sum2/2
  integ1/1 -> Sum1/1, T/1
  Integ2/1 -> T1/1, Sum2/1
  Sum2/1 -> Fcn1/1, Mux/2
  Sum1/1 -> Fcn/1, Mux/1
  signal/1 -> Gain1/1
  Gain1/1 -> Product/2, Product1/1
  Fcn2/1 -> magnitude/1

== system power_wind/Wind Farm/Wind Turbine Protections/Protection System2/AC Voltage Protection/Voltage Measurement/magnitude1/Fourier1 ==
  signal : Inport
  Constant : Constant  Value=0
  Fcn : Fcn  Expr=u^2
  Fcn1 : Fcn  Expr=u^2
  Fcn2 : Fcn  Expr=sqrt(u)
  Fcn3 : Fcn  Expr=180/pi*atan2(u[2],u[1])
  Gain1 : Gain  Gain=k*f1  SaturateOnIntegerOverflow=on  OutDataTypeStr=Inherit: Same as input  ParamDataTypeStr=Inherit: Same as input
  Integ2 : Integrator  InitialConditionSource=external
  Mux : Mux  Inputs=2
  Product : Product  SaturateOnIntegerOverflow=on  InputSameDT=on  OutDataTypeStr=Inherit: Same as first input
  Product1 : Product  SaturateOnIntegerOverflow=on  InputSameDT=on  OutDataTypeStr=Inherit: Same as first input
  Sum : Sum  SaturateOnIntegerOverflow=on  InputSameDT=on  OutDataTypeStr=Inherit: Same as first input
  Sum1 : Sum  Inputs=+-  SaturateOnIntegerOverflow=on  InputSameDT=on  OutDataTypeStr=Inherit: Same as first input
  Sum2 : Sum  Inputs=+-  SaturateOnIntegerOverflow=on  InputSameDT=on  OutDataTypeStr=Inherit: Same as first input
  T : TransportDelay  DelayTime=1/f1  BufferSize=2048
  T1 : TransportDelay  DelayTime=1/f1  BufferSize=2048
  cos(nwt) : Sin  Frequency=2*pi*n*f1  Phase=pi/2  SampleTime=0
  integ1 : Integrator  InitialConditionSource=external
  sin(nwt) : Sin  Frequency=2*pi*n*f1  SampleTime=0
  magnitude : Outport  InitialOutput=0
  angle : Outport  Port=2  InitialOutput=0
  wires:
  Constant/1 -> integ1/2, Integ2/2
  Sum/1 -> Fcn2/1
  Fcn/1 -> Sum/1
  Fcn1/1 -> Sum/2
  Mux/1 -> Fcn3/1
  Fcn3/1 -> angle/1
  sin(nwt)/1 -> Product/1
  cos(nwt)/1 -> Product1/2
  Product/1 -> integ1/1
  Product1/1 -> Integ2/1
  T/1 -> Sum1/2
  T1/1 -> Sum2/2
  integ1/1 -> Sum1/1, T/1
  Integ2/1 -> T1/1, Sum2/1
  Sum2/1 -> Fcn1/1, Mux/2
  Sum1/1 -> Fcn/1, Mux/1
  signal/1 -> Gain1/1
  Gain1/1 -> Product/2, Product1/1
  Fcn2/1 -> magnitude/1

== system power_wind/Wind Farm/Wind Turbine Protections/Protection System2/AC Voltage Protection/Voltage Measurement/magnitude1/Fourier2 ==
  signal : Inport
  Constant : Constant  Value=0
  Fcn : Fcn  Expr=u^2
  Fcn1 : Fcn  Expr=u^2
  Fcn2 : Fcn  Expr=sqrt(u)
  Fcn3 : Fcn  Expr=180/pi*atan2(u[2],u[1])
  Gain1 : Gain  Gain=k*f1  SaturateOnIntegerOverflow=on  OutDataTypeStr=Inherit: Same as input  ParamDataTypeStr=Inherit: Same as input
  Integ2 : Integrator  InitialConditionSource=external
  Mux : Mux  Inputs=2
  Product : Product  SaturateOnIntegerOverflow=on  InputSameDT=on  OutDataTypeStr=Inherit: Same as first input
  Product1 : Product  SaturateOnIntegerOverflow=on  InputSameDT=on  OutDataTypeStr=Inherit: Same as first input
  Sum : Sum  SaturateOnIntegerOverflow=on  InputSameDT=on  OutDataTypeStr=Inherit: Same as first input
  Sum1 : Sum  Inputs=+-  SaturateOnIntegerOverflow=on  InputSameDT=on  OutDataTypeStr=Inherit: Same as first input
  Sum2 : Sum  Inputs=+-  SaturateOnIntegerOverflow=on  InputSameDT=on  OutDataTypeStr=Inherit: Same as first input
  T : TransportDelay  DelayTime=1/f1  BufferSize=2048
  T1 : TransportDelay  DelayTime=1/f1  BufferSize=2048
  cos(nwt) : Sin  Frequency=2*pi*n*f1  Phase=pi/2  SampleTime=0
  integ1 : Integrator  InitialConditionSource=external
  sin(nwt) : Sin  Frequency=2*pi*n*f1  SampleTime=0
  magnitude : Outport  InitialOutput=0
  angle : Outport  Port=2  InitialOutput=0
  wires:
  Fcn2/1 -> magnitude/1
  Gain1/1 -> Product1/1, Product/2
  signal/1 -> Gain1/1
  Sum1/1 -> Mux/1, Fcn/1
  Sum2/1 -> Mux/2, Fcn1/1
  Integ2/1 -> Sum2/1, T1/1
  integ1/1 -> T/1, Sum1/1
  T1/1 -> Sum2/2
  T/1 -> Sum1/2
  Product1/1 -> Integ2/1
  Product/1 -> integ1/1
  cos(nwt)/1 -> Product1/2
  sin(nwt)/1 -> Product/1
  Fcn3/1 -> angle/1
  Mux/1 -> Fcn3/1
  Fcn1/1 -> Sum/2
  Fcn/1 -> Sum/1
  Sum/1 -> Fcn2/1
  Constant/1 -> Integ2/2, integ1/2

== system power_wind/Wind Farm/Wind Turbine Protections/Protection System2/AC Voltage Protection/Voltage Measurement/magnitude2/Fourier1 ==
  signal : Inport
  Constant : Constant  Value=0
  Fcn : Fcn  Expr=u^2
  Fcn1 : Fcn  Expr=u^2
  Fcn2 : Fcn  Expr=sqrt(u)
  Fcn3 : Fcn  Expr=180/pi*atan2(u[2],u[1])
  Gain1 : Gain  Gain=k*f1  SaturateOnIntegerOverflow=on  OutDataTypeStr=Inherit: Same as input  ParamDataTypeStr=Inherit: Same as input
  Integ2 : Integrator  InitialConditionSource=external
  Mux : Mux  Inputs=2
  Product : Product  SaturateOnIntegerOverflow=on  InputSameDT=on  OutDataTypeStr=Inherit: Same as first input
  Product1 : Product  SaturateOnIntegerOverflow=on  InputSameDT=on  OutDataTypeStr=Inherit: Same as first input
  Sum : Sum  SaturateOnIntegerOverflow=on  InputSameDT=on  OutDataTypeStr=Inherit: Same as first input
  Sum1 : Sum  Inputs=+-  SaturateOnIntegerOverflow=on  InputSameDT=on  OutDataTypeStr=Inherit: Same as first input
  Sum2 : Sum  Inputs=+-  SaturateOnIntegerOverflow=on  InputSameDT=on  OutDataTypeStr=Inherit: Same as first input
  T : TransportDelay  DelayTime=1/f1  BufferSize=2048
  T1 : TransportDelay  DelayTime=1/f1  BufferSize=2048
  cos(nwt) : Sin  Frequency=2*pi*n*f1  Phase=pi/2  SampleTime=0
  integ1 : Integrator  InitialConditionSource=external
  sin(nwt) : Sin  Frequency=2*pi*n*f1  SampleTime=0
  magnitude : Outport  InitialOutput=0
  angle : Outport  Port=2  InitialOutput=0
  wires:
  Fcn2/1 -> magnitude/1
  Gain1/1 -> Product1/1, Product/2
  signal/1 -> Gain1/1
  Sum1/1 -> Mux/1, Fcn/1
  Sum2/1 -> Mux/2, Fcn1/1
  Integ2/1 -> Sum2/1, T1/1
  integ1/1 -> T/1, Sum1/1
  T1/1 -> Sum2/2
  T/1 -> Sum1/2
  Product1/1 -> Integ2/1
  Product/1 -> integ1/1
  cos(nwt)/1 -> Product1/2
  sin(nwt)/1 -> Product/1
  Fcn3/1 -> angle/1
  Mux/1 -> Fcn3/1
  Fcn1/1 -> Sum/2
  Fcn/1 -> Sum/1
  Sum/1 -> Fcn2/1
  Constant/1 -> Integ2/2, integ1/2

== system power_wind/Wind Farm/Wind Turbine Protections/Protection System2/AC Voltage Protection/Voltage Measurement/magnitude2/Fourier2 ==
  signal : Inport
  Constant : Constant  Value=0
  Fcn : Fcn  Expr=u^2
  Fcn1 : Fcn  Expr=u^2
  Fcn2 : Fcn  Expr=sqrt(u)
  Fcn3 : Fcn  Expr=180/pi*atan2(u[2],u[1])
  Gain1 : Gain  Gain=k*f1  SaturateOnIntegerOverflow=on  OutDataTypeStr=Inherit: Same as input  ParamDataTypeStr=Inherit: Same as input
  Integ2 : Integrator  InitialConditionSource=external
  Mux : Mux  Inputs=2
  Product : Product  SaturateOnIntegerOverflow=on  InputSameDT=on  OutDataTypeStr=Inherit: Same as first input
  Product1 : Product  SaturateOnIntegerOverflow=on  InputSameDT=on  OutDataTypeStr=Inherit: Same as first input
  Sum : Sum  SaturateOnIntegerOverflow=on  InputSameDT=on  OutDataTypeStr=Inherit: Same as first input
  Sum1 : Sum  Inputs=+-  SaturateOnIntegerOverflow=on  InputSameDT=on  OutDataTypeStr=Inherit: Same as first input
  Sum2 : Sum  Inputs=+-  SaturateOnIntegerOverflow=on  InputSameDT=on  OutDataTypeStr=Inherit: Same as first input
  T : TransportDelay  DelayTime=1/f1  BufferSize=2048
  T1 : TransportDelay  DelayTime=1/f1  BufferSize=2048
  cos(nwt) : Sin  Frequency=2*pi*n*f1  Phase=pi/2  SampleTime=0
  integ1 : Integrator  InitialConditionSource=external
  sin(nwt) : Sin  Frequency=2*pi*n*f1  SampleTime=0
  magnitude : Outport  InitialOutput=0
  angle : Outport  Port=2  InitialOutput=0
  wires:
  Constant/1 -> integ1/2, Integ2/2
  Sum/1 -> Fcn2/1
  Fcn/1 -> Sum/1
  Fcn1/1 -> Sum/2
  Mux/1 -> Fcn3/1
  Fcn3/1 -> angle/1
  sin(nwt)/1 -> Product/1
  cos(nwt)/1 -> Product1/2
  Product/1 -> integ1/1
  Product1/1 -> Integ2/1
  T/1 -> Sum1/2
  T1/1 -> Sum2/2
  integ1/1 -> Sum1/1, T/1
  Integ2/1 -> T1/1, Sum2/1
  Sum2/1 -> Fcn1/1, Mux/2
  Sum1/1 -> Fcn/1, Mux/1
  signal/1 -> Gain1/1
  Gain1/1 -> Product/2, Product1/1
  Fcn2/1 -> magnitude/1

== system power_wind/Wind Farm/Wind Turbine Protections/Protection System3/AC Current Protection/Current Measurement/magnitude/Fourier1 ==
  signal : Inport
  Constant : Constant  Value=0
  Fcn : Fcn  Expr=u^2
  Fcn1 : Fcn  Expr=u^2
  Fcn2 : Fcn  Expr=sqrt(u)
  Fcn3 : Fcn  Expr=180/pi*atan2(u[2],u[1])
  Gain1 : Gain  Gain=k*f1  SaturateOnIntegerOverflow=on  OutDataTypeStr=Inherit: Same as input  ParamDataTypeStr=Inherit: Same as input
  Integ2 : Integrator  InitialConditionSource=external
  Mux : Mux  Inputs=2
  Product : Product  SaturateOnIntegerOverflow=on  InputSameDT=on  OutDataTypeStr=Inherit: Same as first input
  Product1 : Product  SaturateOnIntegerOverflow=on  InputSameDT=on  OutDataTypeStr=Inherit: Same as first input
  Sum : Sum  SaturateOnIntegerOverflow=on  InputSameDT=on  OutDataTypeStr=Inherit: Same as first input
  Sum1 : Sum  Inputs=+-  SaturateOnIntegerOverflow=on  InputSameDT=on  OutDataTypeStr=Inherit: Same as first input
  Sum2 : Sum  Inputs=+-  SaturateOnIntegerOverflow=on  InputSameDT=on  OutDataTypeStr=Inherit: Same as first input
  T : TransportDelay  DelayTime=1/f1  BufferSize=2048
  T1 : TransportDelay  DelayTime=1/f1  BufferSize=2048
  cos(nwt) : Sin  Frequency=2*pi*n*f1  Phase=pi/2  SampleTime=0
  integ1 : Integrator  InitialConditionSource=external
  sin(nwt) : Sin  Frequency=2*pi*n*f1  SampleTime=0
  magnitude : Outport  InitialOutput=0
  angle : Outport  Port=2  InitialOutput=0
  wires:
  Constant/1 -> integ1/2, Integ2/2
  Sum/1 -> Fcn2/1
  Fcn/1 -> Sum/1
  Fcn1/1 -> Sum/2
  Mux/1 -> Fcn3/1
  Fcn3/1 -> angle/1
  sin(nwt)/1 -> Product/1
  cos(nwt)/1 -> Product1/2
  Product/1 -> integ1/1
  Product1/1 -> Integ2/1
  T/1 -> Sum1/2
  T1/1 -> Sum2/2
  integ1/1 -> Sum1/1, T/1
  Integ2/1 -> T1/1, Sum2/1
  Sum2/1 -> Fcn1/1, Mux/2
  Sum1/1 -> Fcn/1, Mux/1
  signal/1 -> Gain1/1
  Gain1/1 -> Product/2, Product1/1
  Fcn2/1 -> magnitude/1

== system power_wind/Wind Farm/Wind Turbine Protections/Protection System3/AC Current Protection/Current Measurement/magnitude/Fourier2 ==
  signal : Inport
  Constant : Constant  Value=0
  Fcn : Fcn  Expr=u^2
  Fcn1 : Fcn  Expr=u^2
  Fcn2 : Fcn  Expr=sqrt(u)
  Fcn3 : Fcn  Expr=180/pi*atan2(u[2],u[1])
  Gain1 : Gain  Gain=k*f1  SaturateOnIntegerOverflow=on  OutDataTypeStr=Inherit: Same as input  ParamDataTypeStr=Inherit: Same as input
  Integ2 : Integrator  InitialConditionSource=external
  Mux : Mux  Inputs=2
  Product : Product  SaturateOnIntegerOverflow=on  InputSameDT=on  OutDataTypeStr=Inherit: Same as first input
  Product1 : Product  SaturateOnIntegerOverflow=on  InputSameDT=on  OutDataTypeStr=Inherit: Same as first input
  Sum : Sum  SaturateOnIntegerOverflow=on  InputSameDT=on  OutDataTypeStr=Inherit: Same as first input
  Sum1 : Sum  Inputs=+-  SaturateOnIntegerOverflow=on  InputSameDT=on  OutDataTypeStr=Inherit: Same as first input
  Sum2 : Sum  Inputs=+-  SaturateOnIntegerOverflow=on  InputSameDT=on  OutDataTypeStr=Inherit: Same as first input
  T : TransportDelay  DelayTime=1/f1  BufferSize=2048
  T1 : TransportDelay  DelayTime=1/f1  BufferSize=2048
  cos(nwt) : Sin  Frequency=2*pi*n*f1  Phase=pi/2  SampleTime=0
  integ1 : Integrator  InitialConditionSource=external
  sin(nwt) : Sin  Frequency=2*pi*n*f1  SampleTime=0
  magnitude : Outport  InitialOutput=0
  angle : Outport  Port=2  InitialOutput=0
  wires:
  Fcn2/1 -> magnitude/1
  Gain1/1 -> Product1/1, Product/2
  signal/1 -> Gain1/1
  Sum1/1 -> Mux/1, Fcn/1
  Sum2/1 -> Mux/2, Fcn1/1
  Integ2/1 -> Sum2/1, T1/1
  integ1/1 -> T/1, Sum1/1
  T1/1 -> Sum2/2
  T/1 -> Sum1/2
  Product1/1 -> Integ2/1
  Product/1 -> integ1/1
  cos(nwt)/1 -> Product1/2
  sin(nwt)/1 -> Product/1
  Fcn3/1 -> angle/1
  Mux/1 -> Fcn3/1
  Fcn1/1 -> Sum/2
  Fcn/1 -> Sum/1
  Sum/1 -> Fcn2/1
  Constant/1 -> Integ2/2, integ1/2

== system power_wind/Wind Farm/Wind Turbine Protections/Protection System3/AC Current Protection/Current Measurement/magnitude1/Fourier1 ==
  signal : Inport
  Constant : Constant  Value=0
  Fcn : Fcn  Expr=u^2
  Fcn1 : Fcn  Expr=u^2
  Fcn2 : Fcn  Expr=sqrt(u)
  Fcn3 : Fcn  Expr=180/pi*atan2(u[2],u[1])
  Gain1 : Gain  Gain=k*f1  SaturateOnIntegerOverflow=on  OutDataTypeStr=Inherit: Same as input  ParamDataTypeStr=Inherit: Same as input
  Integ2 : Integrator  InitialConditionSource=external
  Mux : Mux  Inputs=2
  Product : Product  SaturateOnIntegerOverflow=on  InputSameDT=on  OutDataTypeStr=Inherit: Same as first input
  Product1 : Product  SaturateOnIntegerOverflow=on  InputSameDT=on  OutDataTypeStr=Inherit: Same as first input
  Sum : Sum  SaturateOnIntegerOverflow=on  InputSameDT=on  OutDataTypeStr=Inherit: Same as first input
  Sum1 : Sum  Inputs=+-  SaturateOnIntegerOverflow=on  InputSameDT=on  OutDataTypeStr=Inherit: Same as first input
  Sum2 : Sum  Inputs=+-  SaturateOnIntegerOverflow=on  InputSameDT=on  OutDataTypeStr=Inherit: Same as first input
  T : TransportDelay  DelayTime=1/f1  BufferSize=2048
  T1 : TransportDelay  DelayTime=1/f1  BufferSize=2048
  cos(nwt) : Sin  Frequency=2*pi*n*f1  Phase=pi/2  SampleTime=0
  integ1 : Integrator  InitialConditionSource=external
  sin(nwt) : Sin  Frequency=2*pi*n*f1  SampleTime=0
  magnitude : Outport  InitialOutput=0
  angle : Outport  Port=2  InitialOutput=0
  wires:
  Fcn2/1 -> magnitude/1
  Gain1/1 -> Product1/1, Product/2
  signal/1 -> Gain1/1
  Sum1/1 -> Mux/1, Fcn/1
  Sum2/1 -> Mux/2, Fcn1/1
  Integ2/1 -> Sum2/1, T1/1
  integ1/1 -> T/1, Sum1/1
  T1/1 -> Sum2/2
  T/1 -> Sum1/2
  Product1/1 -> Integ2/1
  Product/1 -> integ1/1
  cos(nwt)/1 -> Product1/2
  sin(nwt)/1 -> Product/1
  Fcn3/1 -> angle/1
  Mux/1 -> Fcn3/1
  Fcn1/1 -> Sum/2
  Fcn/1 -> Sum/1
  Sum/1 -> Fcn2/1
  Constant/1 -> Integ2/2, integ1/2

== system power_wind/Wind Farm/Wind Turbine Protections/Protection System3/AC Current Protection/Current Measurement/magnitude1/Fourier2 ==
  signal : Inport
  Constant : Constant  Value=0
  Fcn : Fcn  Expr=u^2
  Fcn1 : Fcn  Expr=u^2
  Fcn2 : Fcn  Expr=sqrt(u)
  Fcn3 : Fcn  Expr=180/pi*atan2(u[2],u[1])
  Gain1 : Gain  Gain=k*f1  SaturateOnIntegerOverflow=on  OutDataTypeStr=Inherit: Same as input  ParamDataTypeStr=Inherit: Same as input
  Integ2 : Integrator  InitialConditionSource=external
  Mux : Mux  Inputs=2
  Product : Product  SaturateOnIntegerOverflow=on  InputSameDT=on  OutDataTypeStr=Inherit: Same as first input
  Product1 : Product  SaturateOnIntegerOverflow=on  InputSameDT=on  OutDataTypeStr=Inherit: Same as first input
  Sum : Sum  SaturateOnIntegerOverflow=on  InputSameDT=on  OutDataTypeStr=Inherit: Same as first input
  Sum1 : Sum  Inputs=+-  SaturateOnIntegerOverflow=on  InputSameDT=on  OutDataTypeStr=Inherit: Same as first input
  Sum2 : Sum  Inputs=+-  SaturateOnIntegerOverflow=on  InputSameDT=on  OutDataTypeStr=Inherit: Same as first input
  T : TransportDelay  DelayTime=1/f1  BufferSize=2048
  T1 : TransportDelay  DelayTime=1/f1  BufferSize=2048
  cos(nwt) : Sin  Frequency=2*pi*n*f1  Phase=pi/2  SampleTime=0
  integ1 : Integrator  InitialConditionSource=external
  sin(nwt) : Sin  Frequency=2*pi*n*f1  SampleTime=0
  magnitude : Outport  InitialOutput=0
  angle : Outport  Port=2  InitialOutput=0
  wires:
  Constant/1 -> integ1/2, Integ2/2
  Sum/1 -> Fcn2/1
  Fcn/1 -> Sum/1
  Fcn1/1 -> Sum/2
  Mux/1 -> Fcn3/1
  Fcn3/1 -> angle/1
  sin(nwt)/1 -> Product/1
  cos(nwt)/1 -> Product1/2
  Product/1 -> integ1/1
  Product1/1 -> Integ2/1
  T/1 -> Sum1/2
  T1/1 -> Sum2/2
  integ1/1 -> Sum1/1, T/1
  Integ2/1 -> T1/1, Sum2/1
  Sum2/1 -> Fcn1/1, Mux/2
  Sum1/1 -> Fcn/1, Mux/1
  signal/1 -> Gain1/1
  Gain1/1 -> Product/2, Product1/1
  Fcn2/1 -> magnitude/1
